simulink model "g_position_control"  (R2024b)
settings: Solver=VariableStepAuto  StartTime=0.0  StopTime=10.0  RelTol=1e-3
settings Model: Creator=Hp  LastModifiedBy=Hp

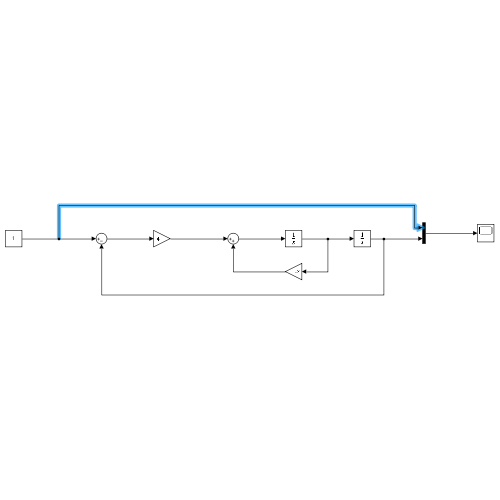
[thumbnail: Simulink's stored preview of the top-level diagram]
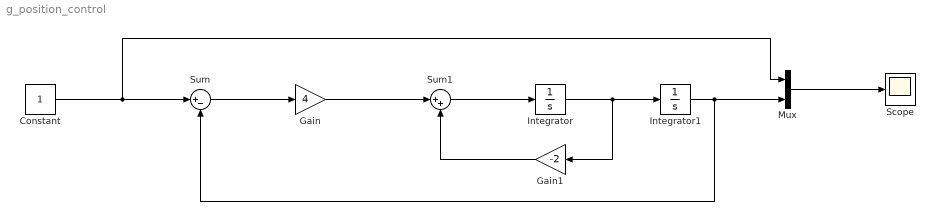
== system g_position_control ==
  Constant : Constant
  Gain : Gain  Gain=4
  Gain1 : Gain  Gain=-2
  Integrator : Integrator
  Integrator1 : Integrator
  Mux : Mux  Inputs=2
  Scope : Scope
  Sum : Sum  Inputs=|+-
  Sum1 : Sum  Inputs=|++
  wires:
  Constant/1 -> Mux/1, Sum/1
  Sum/1 -> Gain/1
  Gain/1 -> Sum1/1
  Integrator/1 -> Gain1/1, Integrator1/1
  Sum1/1 -> Integrator/1
  Gain1/1 -> Sum1/2
  Integrator1/1 -> Sum/2, Mux/2
  Mux/1 -> Scope/1
